simulink model "LIA"  (R2022b)
settings: Solver=VariableStepAuto  StartTime=0.0  StopTime=10.0  RelTol=1e-3
libraries: dsparch4 x2, dspswit3 x1
settings Model: Creator=zhang  LastModifiedBy=zhang

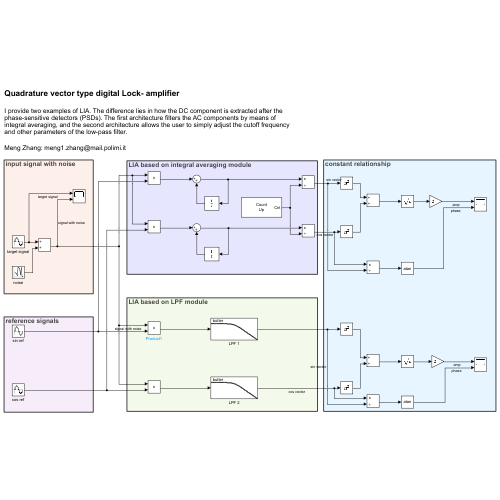
[thumbnail: Simulink's stored preview of the top-level diagram]
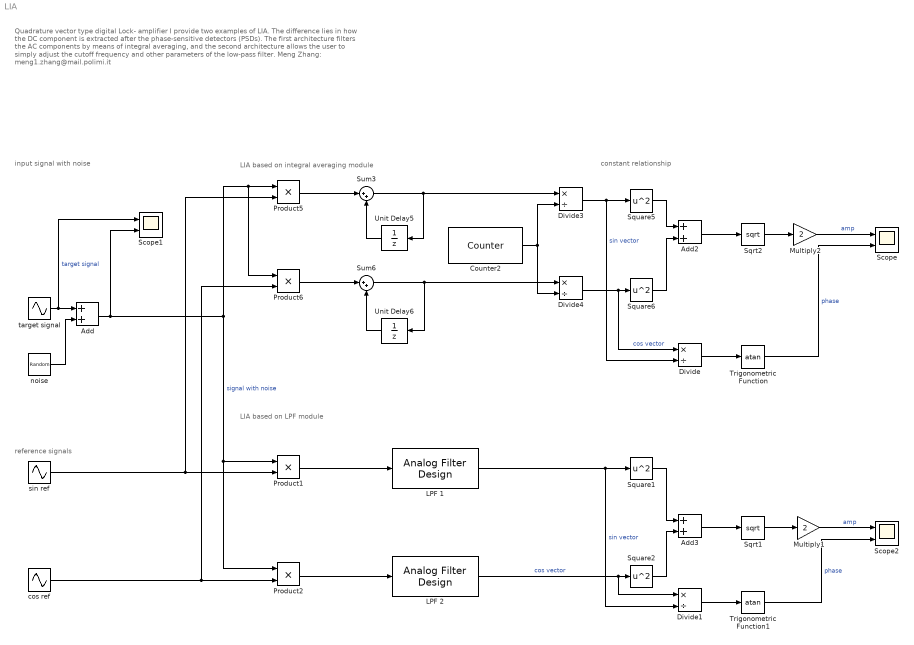
== system LIA ==
  note: Quadrature vector type digital Lock- amplifier
      |
      | I provide two examples of LIA. The difference lies in how the DC component is extracted after the phase-sensitive detectors (PSDs). The first architecture filters the AC components by means of integral averaging, and the second architecture allows the user to simply adjust the cutoff frequency and other parameters of the low-pass filter.
      |
      | Meng Zhang: meng1.zhang@mail.polimi.it
  note: input signal with noise
  note: reference signals
  note: LIA based on integral averaging module
  note: LIA based on LPF module
  note: constant relationship
  Add : Sum
  Add2 : Sum
  Add3 : Sum
  Counter2 : dspswit3/Counter  Direction=Up  CountEvent=Free running  CounterSize=32 bits  MaxCount=255  InitialCount=1  Output=Count  HitValue=32  ResetInput=off  SamplesPerFrame=1  Ts=1/12000  CntDtype=single  HitDtype=Logical
  Divide{,1,3..4} (4 alike) : Product  Inputs=*/
  LPF 1 : dsparch4/Analog Filter Design  method=Butterworth  filttype=Lowpass  N=2  Wlo=5  Whi=80  Rp=2  Rs=40
  LPF 2 : dsparch4/Analog Filter Design  method=Butterworth  filttype=Lowpass  N=2  Wlo=5  Whi=80  Rp=2  Rs=40
  Multiply1 : Gain  Gain=2
  Multiply2 : Gain  Gain=2
  Product{1..2,5..6} (4 alike) : Product
  Scope : Scope  NumInputPorts=2
  Scope1 : Scope  NumInputPorts=2
  Scope2 : Scope  NumInputPorts=2
  Sqrt1 : Sqrt
  Sqrt2 : Sqrt
  Square{1..2,5..6} (4 alike) : Math  Operator=square  SignedPower=on
  Sum3 : Sum  Inputs=|++
  Sum6 : Sum  Inputs=|++
  Trigonometric Function : Trigonometry  Operator=atan
  Trigonometric Function1 : Trigonometry  Operator=atan
  Unit Delay5 : UnitDelay  SampleTime=-1  HasFrameUpgradeWarning=on
  Unit Delay6 : UnitDelay  SampleTime=-1  HasFrameUpgradeWarning=on
  cos ref : Sin  Frequency=50  Phase=0.5*pi  SampleTime=1/12000
  noise : RandomNumber  Variance=10  SampleTime=1/12000
  sin ref : Sin  Frequency=50  SampleTime=1/12000
  target signal : Sin  Frequency=50  Phase=0.3*pi  SampleTime=1/12000
  wires:
  Unit Delay6/1 -> Sum6/2
  Multiply2/1 -> Scope/1  "amp"
  Sum3/1 -> Unit Delay5/1, Divide3/1
  Add2/1 -> Sqrt2/1
  Sum6/1 -> Divide4/1, Unit Delay6/1
  Counter2/1 -> Divide4/2, Divide3/2
  Square5/1 -> Add2/1
  Divide3/1 -> Divide/2, Square5/1  "sin vector"
  Sqrt2/1 -> Multiply2/1
  Product5/1 -> Sum3/1
  Unit Delay5/1 -> Sum3/2
  Product6/1 -> Sum6/1
  Square6/1 -> Add2/2
  Divide4/1 -> Divide/1, Square6/1  "cos vector"
  target signal/1 -> Scope1/1, Add/1  "target signal"
  noise/1 -> Add/2
  Divide/1 -> Trigonometric Function/1
  Trigonometric Function/1 -> Scope/2  "phase"
  Add/1 -> Product5/1, Product6/1, Product2/1, Product1/1, Scope1/2  "signal with noise"
  Multiply1/1 -> Scope2/1  "amp"
  cos ref/1 -> Product6/2, Product2/2
  Divide1/1 -> Trigonometric Function1/1
  Sqrt1/1 -> Multiply1/1
  LPF 1/1 -> Divide1/2, Square1/1  "sin vector"
  LPF 2/1 -> Square2/1, Divide1/1  "cos vector"
  Trigonometric Function1/1 -> Scope2/2  "phase"
  sin ref/1 -> Product5/2, Product1/2
  Square1/1 -> Add3/1
  Square2/1 -> Add3/2
  Add3/1 -> Sqrt1/1
  Product2/1 -> LPF 2/1
  Product1/1 -> LPF 1/1
